simulink model "svpwm_induction_motor"  (R2023b)
settings: Solver=FixedStepAuto  StartTime=0  StopTime=2  FixedStep=1e-5  RelTol=1e-3
libraries: slpidlib x3, spsAsynchronousMachineSIUnitsLib x1, spsDCVoltageSourceLib x1, simulink x1, spsabctodq0Lib x1, spsdq0toAlphaBetaZeroLib x1, spsThreePhaseVIMeasurementLib x1, spsUniversalBridgeLib x1, spspowerguiLib x1
settings Model: Creator=朱子轩  LastModifiedBy=13571

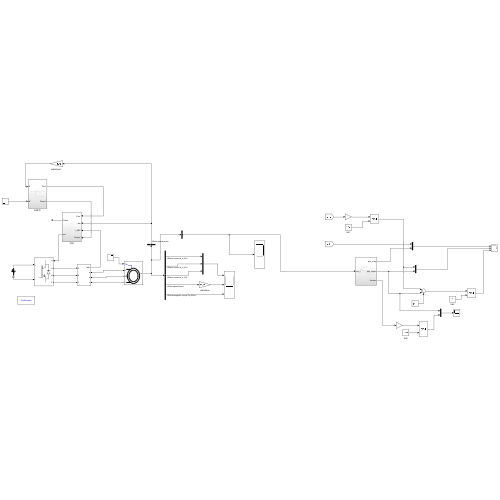
[thumbnail: Simulink's stored preview of the top-level diagram]
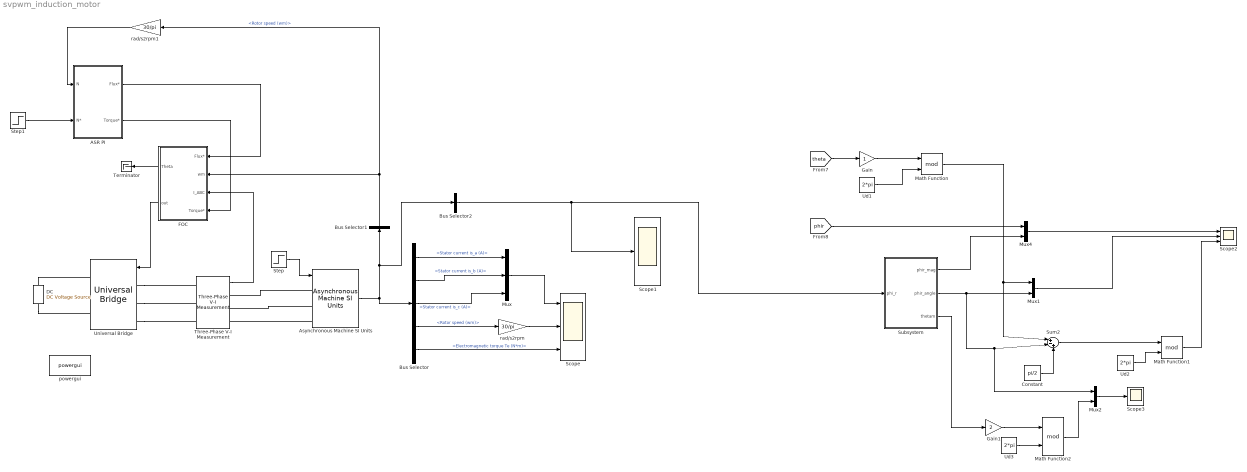
== system svpwm_induction_motor ==
  ASR PI : Subsystem
  Asynchronous Machine SI Units : spsAsynchronousMachineSIUnitsLib/Asynchronous Machine SI Units  RotorType=Squirrel-cage  PresetModel=No  MechanicalLoad=Torque Tm  ShowDetailedParameters=on  ReferenceFrame=Stationary  Units=SI  MeasurementBus=off  NominalParameters=[7500,380,50]  VoltageRatio=1  Stator=[0.7384,0.003045]  Rotor=[0.7402,0.003045]  Cage1=[0.4155 0.002066]  Cage2=[0.4168 0.0003495]  Lm=0.1241  Mechanical=[0.0343,0,2]  PolePairs=2  InitialConditions=[1,0,0,0,0,0,0,0]  SimulateSaturation=off  Saturation=[14.03593122, 27.81365428, 53.79336849, 72.68890987, 97.98006896, 148.6815601, 215.7428561, 302.9841135, 428.7778367 ; 230, 322, 414, 460, 506, 552, 598, 644, 690]  LoadFlowParameters=1492000  TsPowergui=0  TsBlock=-1  IterativeModel=Trapezoidal non iterative  IterativeDiscreteModel=Trapezoidal non iterative  Pmec=1.492e+006
  Bus Selector : BusSelector  OutputSignals=Stator measurements.Stator current is_a (A),Stator measurements.Stator current is_b (A),Stator measurements.Stator current is_c (A),Mechanical.Rotor speed (wm),Mechanical.Electromagnetic torque Te (N*m)
  Bus Selector1 : BusSelector  OutputSignals=Mechanical.Rotor speed (wm)
  Bus Selector2 : BusSelector  OutputSignals=Rotor measurements.Rotor flux phir_d (V s),Rotor measurements.Rotor flux phir_q (V s),Mechanical.Rotor angle thetam (rad)  OutputAsBus=on
  Constant : Constant  Value=pi/2
  DC : spsDCVoltageSourceLib/DC Voltage Source  Amplitude=800  Measurements=None
  FOC : Subsystem
  Gain : Gain
  Gain1 : Gain  Gain=2
  Math Function : Math  Operator=mod
  Math Function1 : Math  Operator=mod
  Math Function2 : Math  Operator=mod
  Mux : Mux  Inputs=3
  Mux1 : Mux  Inputs=2
  Mux2 : Mux  Inputs=2
  Mux4 : Mux  Inputs=2
  Scope : Scope  NumInputPorts=3
  Scope1 : Scope
  Scope2 : Scope  NumInputPorts=3
  Scope3 : Scope
  Step : Step  Time=0.5  After=40  SampleTime=0
  Step1 : Step  Before=1000  After=1400  SampleTime=0
  Subsystem : Subsystem
  Sum2 : Sum  Inputs=|+-+
  Terminator : Terminator
  Three-Phase V-I Measurement : spsThreePhaseVIMeasurementLib/Three-Phase V-I Measurement  VoltageMeasurement=no  SetLabelV=off  LabelV=Vabc  Vpu=off  VpuLL=off  CurrentMeasurement=yes  SetLabelI=off  LabelI=Iabc  Ipu=off  Pbase=100e6  Vbase=500e3  OutputType=Complex  PhasorSimulation=off  PSBequivalent=0
  Ud1 : Constant  Value=2*pi
  Ud2 : Constant  Value=2*pi
  Ud3 : Constant  Value=2*pi
  Universal Bridge : spsUniversalBridgeLib/Universal Bridge  Arms=3  SnubberResistance=1e5  SnubberCapacitance=inf  Device=IGBT / Diodes  Ron=1e-3  Lon=0  ForwardVoltages="[  0  0  ]"  ForwardVoltage=0  GTOparameters=[ 10e-6 , 20e-6 ]  IGBTparameters=[ 1e-6 , 2e-6 ]  Measurements=None  Measurements_2=None  converterType=Rectifier
  powergui : spspowerguiLib/powergui  Priority=1  SimulationMode=Continuous  SampleTime=50e-6  frequency=60  Iterations=50  frequencyindice=50  Pbase=100e6  ErrMax=1e-4  UnitsV=kV  UnitsW=MW  buscounter=0  FunctionMessages=off  echomessages=off  EnableUseOfTLC=off  CurrentSourceSwitches=off  DisableSnubberDevices=off  DisableRonSwitches=off  DisableVfSwitches=off  DisplayEquations=off  AutomaticDiscreteSolvers=off  SolverType=Tustin/Backward Euler (TBE)  Interpol=off  ExternalGateDelay=off  methode=off  Ts=100  x0status=blocks  SPID=on  SwTol=0  HookPort=off  NonlinearTolerance=1e-4  nMaxIteration=100  ContinueOnMaxIteration=off  RestoreLinks=warning  ResistiveCurrentMeasurement=off  Frange=[0:2:500]  Ylog=off  Xlog=on  ShowGrid=off  save=off  variable=ZData  structure=0  ZoomFFT=off  StartTime=0.0  cycles=1  DisplayStyle=1  fundamental=60  FreqAxis=off  MaxFrequency=1000  frequencyindicesteady=1  RmsSteady=1  display=off
  rad/s2rpm : Gain  Gain=30/pi
  rad/s2rpm1 : Gain  Gain=30/pi
  wires:
  Step/1 -> Asynchronous Machine SI Units/1
  Asynchronous Machine SI Units/1 -> Bus Selector/1, Bus Selector2/1, Bus Selector1/1
  Bus Selector/1 -> Mux/1  "<Stator current is_a (A)>"
  Bus Selector/2 -> Mux/2  "<Stator current is_b (A)>"
  Bus Selector/3 -> Mux/3  "<Stator current is_c (A)>"
  Bus Selector/4 -> rad/s2rpm/1  "<Rotor speed (wm)>"
  Mux/1 -> Scope/1
  rad/s2rpm/1 -> Scope/2
  Step1/1 -> ASR PI/2(N*)
  Bus Selector1/1 -> FOC/2(wm), rad/s2rpm1/1  "<Rotor speed (wm)>"
  rad/s2rpm1/1 -> ASR PI/1(N)
  Three-Phase V-I Measurement/1 -> FOC/3(I_ABC)
  ASR PI/2(Torque*) -> FOC/4(Torque*)
  ASR PI/1(Flux*) -> FOC/1(Flux*)
  FOC/2(out) -> Universal Bridge/1
  Bus Selector2/1 -> Subsystem/1(phi_r), Scope1/1
  Bus Selector/5 -> Scope/3  "<Electromagnetic torque Te (N*m)>"
  FOC/1(Theta) -> Terminator/1
  Ud1/1 -> Math Function/2
  Ud2/1 -> Math Function1/2
  Sum2/1 -> Math Function1/1
  Subsystem/1(phir_mag) -> Mux4/2
  Gain1/1 -> Math Function2/1
  Ud3/1 -> Math Function2/2
  Gain/1 -> Math Function/1
  Mux2/1 -> Scope3/1
  Math Function2/1 -> Mux2/2
  Constant/1 -> Sum2/3
  [theta] -> Gain/1
  [phir] -> Mux4/1
  Mux4/1 -> Scope2/1
  Mux1/1 -> Scope2/2
  Subsystem/2(phir_angle) -> Mux1/2, Mux2/1, Sum2/2
  Subsystem/3(thetam) -> Gain1/1
  Math Function/1 -> Mux1/1, Sum2/1
  Math Function1/1 -> Scope2/3
  connections:
  DC/RConn1 -- Universal Bridge/RConn1
  Universal Bridge/LConn1 -- Three-Phase V-I Measurement/LConn1
  Universal Bridge/LConn2 -- Three-Phase V-I Measurement/LConn2
  Universal Bridge/LConn3 -- Three-Phase V-I Measurement/LConn3
  Asynchronous Machine SI Units/LConn3 -- Three-Phase V-I Measurement/RConn3
  Asynchronous Machine SI Units/LConn2 -- Three-Phase V-I Measurement/RConn2
  Asynchronous Machine SI Units/LConn1 -- Three-Phase V-I Measurement/RConn1
  DC/LConn1 -- Universal Bridge/RConn2

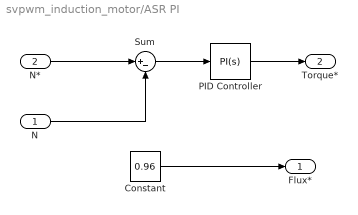
== system svpwm_induction_motor/ASR PI ==
  N : Inport
  N* : Inport  Port=2
  Constant : Constant  Value=0.96
  PID Controller : slpidlib/PID Controller  Controller=PI  Form=Parallel  TimeDomain=Continuous-time  UseExternalTs=off  SampleTime=-1  IntegratorMethod=Forward Euler  FilterMethod=Forward Euler  ControllerParametersSource=internal  P=10  I=10  UseKiTs=off  D=0  N=100  UseFilter=on  TunerSelectOption=Transfer Function Based (PID Tuner App)  InitialConditionSource=internal  InitialConditionForIntegrator=0  InitialConditionForFilter=0  DifferentiatorICPrevScaledInput=0  ExternalReset=none  TrackingMode=off  Kt=1  LimitOutput=on  SatLimitsSource=internal  UpperSaturationLimit=100  LowerSaturationLimit=-100  LinearizeAsGain=on  AntiWindupMode=back-calculation  Kb=1  LimitIntegrator=off  UpperIntegratorSaturationLimit=inf  LowerIntegratorSaturationLimit=-inf  POutMin=[]  POutMax=[]  IOutMin=[]  IOutMax=[]  DOutMin=[]  DOutMax=[]  NOutMin=[]  NOutMax=[]  SumOutMin=[]  SumOutMax=[]  SaturationOutMin=[]  SaturationOutMax=[]  PParamMin=[]  PParamMax=[]  IParamMin=[]  IParamMax=[]  DParamMin=[]  DParamMax=[]  NParamMin=[]  NParamMax=[]  KbParamMin=[]  KbParamMax=[]  KtParamMin=[]  KtParamMax=[]  KbOutMin=[]  KbOutMax=[]  KtOutMin=[]  KtOutMax=[]  IntegratorOutMin=[]  IntegratorOutMax=[]  FilterOutMin=[]  FilterOutMax=[]  SumI1OutMin=[]  SumI1OutMax=[]  SumI2OutMin=[]  SumI2OutMax=[]  SumI3OutMin=[]  SumI3OutMax=[]  SumI4OutMin=[]  SumI4OutMax=[]  SumDOutMin=[]  SumDOutMax=[]  DifferentiatorOutMin=[]  DifferentiatorOutMax=[]  FilterDiffOutCoefMin=[]  FilterDiffOutCoefMax=[]  ReciprocalOutMin=[]  ReciprocalOutMax=[]  SumDenOutMin=[]  SumDenOutMax=[]  SumNumOutMin=[]  SumNumOutMax=[]  DivideOutMin=[]  DivideOutMax=[]  UdiffTsProdOutMin=[]  UdiffTsProdOutMax=[]  NTsProdOutMin=[]  NTsProdOutMax=[]  UintegralTsProdOutMin=[]  UintegralTsProdOutMax=[]  UngainTsProdOutMin=[]  UngainTsProdOutMax=[]  ClampingZeroOutDataTypeStr=Inherit: Inherit via back propagation  ClampingZeroOutMin=[]  ClampingZeroOutMax=[]  FilterDenConstantOutDataTypeStr=Inherit: Inherit via back propagation  FilterDenConstantOutMin=[]  FilterDenConstantOutMax=[]  PCopyOutDataTypeStr=Inherit: Inherit via back propagation  PCopyOutMin=[]  PCopyOutMax=[]  NCopyOutDataTypeStr=Inherit: Inherit via back propagation  NCopyOutMin=[]  NCopyOutMax=[]  IntegratorContinuousStateAttributes=''  IntegratorStateMustResolveToSignalObject=off  IntegratorRTWStateStorageClass=Auto  FilterContinuousStateAttributes=''  FilterStateMustResolveToSignalObject=off  FilterRTWStateStorageClass=Auto  ParallelPVariant=InternalParameters  IdealPVariant=Disabled  IVariant=InternalParameters  DVariant=Disabled  IntegratorVariant=Continuous  SatVariant=Enabled  AWVariant=BackCalculation  PCopyVariant=Disabled  TRVariant=Disabled  FdbkBlocksVariant=Forward  IdealPFdbkVariant=Disabled  SatFdbkVariant=Disabled  DerivativeFilterVariant=Disabled  NVariant=Disabled  NCopyVariant=Disabled_SignalSpec  FilterICVariant=Disabled  IntegratorICVariant=InternalICs  ExternalResetVariant=Disabled  TRSumVariant=Passthrough  SumFdbkVariant=Disabled  SumVariant=Sum_PI  TsampFilterVariant=InternalTs  TsampNgainVariant=Passthrough  TsampIntegralVariant=Disabled_SignalSpec  ExternalSaturationOutDataTypeStr=Inherit: Same as second input
  Sum : Sum  Inputs=|+-
  Flux* : Outport
  Torque* : Outport  Port=2
  wires:
  N*/1 -> Sum/1
  N/1 -> Sum/2
  Constant/1 -> Flux*/1
  Sum/1 -> PID Controller/1
  PID Controller/1 -> Torque*/1

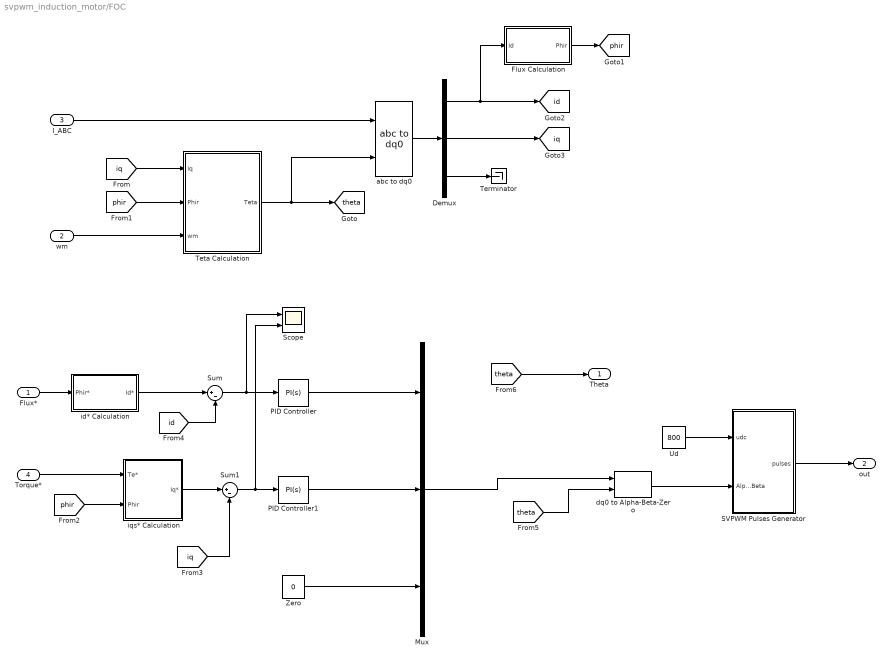
== system svpwm_induction_motor/FOC ==
  Flux* : Inport
  wm : Inport  Port=2
  I_ABC : Inport  Port=3
  Torque* : Inport  Port=4
  Demux : Demux  Outputs=3
  Flux Calculation : Subsystem
  Mux : Mux  Inputs=3
  PID Controller : slpidlib/PID Controller  Controller=PI  Form=Parallel  TimeDomain=Continuous-time  UseExternalTs=off  SampleTime=-1  IntegratorMethod=Forward Euler  FilterMethod=Forward Euler  ControllerParametersSource=internal  P=100  I=1  UseKiTs=off  D=0  N=100  UseFilter=on  TunerSelectOption=Transfer Function Based (PID Tuner App)  InitialConditionSource=internal  InitialConditionForIntegrator=0  InitialConditionForFilter=0  DifferentiatorICPrevScaledInput=0  ExternalReset=none  TrackingMode=off  Kt=1  LimitOutput=off  SatLimitsSource=internal  UpperSaturationLimit=100  LowerSaturationLimit=-100  LinearizeAsGain=on  AntiWindupMode=back-calculation  Kb=1  LimitIntegrator=off  UpperIntegratorSaturationLimit=inf  LowerIntegratorSaturationLimit=-inf  POutMin=[]  POutMax=[]  IOutMin=[]  IOutMax=[]  DOutMin=[]  DOutMax=[]  NOutMin=[]  NOutMax=[]  SumOutMin=[]  SumOutMax=[]  SaturationOutMin=[]  SaturationOutMax=[]  PParamMin=[]  PParamMax=[]  IParamMin=[]  IParamMax=[]  DParamMin=[]  DParamMax=[]  NParamMin=[]  NParamMax=[]  KbParamMin=[]  KbParamMax=[]  KtParamMin=[]  KtParamMax=[]  KbOutMin=[]  KbOutMax=[]  KtOutMin=[]  KtOutMax=[]  IntegratorOutMin=[]  IntegratorOutMax=[]  FilterOutMin=[]  FilterOutMax=[]  SumI1OutMin=[]  SumI1OutMax=[]  SumI2OutMin=[]  SumI2OutMax=[]  SumI3OutMin=[]  SumI3OutMax=[]  SumI4OutMin=[]  SumI4OutMax=[]  SumDOutMin=[]  SumDOutMax=[]  DifferentiatorOutMin=[]  DifferentiatorOutMax=[]  FilterDiffOutCoefMin=[]  FilterDiffOutCoefMax=[]  ReciprocalOutMin=[]  ReciprocalOutMax=[]  SumDenOutMin=[]  SumDenOutMax=[]  SumNumOutMin=[]  SumNumOutMax=[]  DivideOutMin=[]  DivideOutMax=[]  UdiffTsProdOutMin=[]  UdiffTsProdOutMax=[]  NTsProdOutMin=[]  NTsProdOutMax=[]  UintegralTsProdOutMin=[]  UintegralTsProdOutMax=[]  UngainTsProdOutMin=[]  UngainTsProdOutMax=[]  ClampingZeroOutDataTypeStr=Inherit: Inherit via back propagation  ClampingZeroOutMin=[]  ClampingZeroOutMax=[]  FilterDenConstantOutDataTypeStr=Inherit: Inherit via back propagation  FilterDenConstantOutMin=[]  FilterDenConstantOutMax=[]  PCopyOutDataTypeStr=Inherit: Inherit via back propagation  PCopyOutMin=[]  PCopyOutMax=[]  NCopyOutDataTypeStr=Inherit: Inherit via back propagation  NCopyOutMin=[]  NCopyOutMax=[]  IntegratorContinuousStateAttributes=''  IntegratorStateMustResolveToSignalObject=off  IntegratorRTWStateStorageClass=Auto  FilterContinuousStateAttributes=''  FilterStateMustResolveToSignalObject=off  FilterRTWStateStorageClass=Auto  ParallelPVariant=InternalParameters  IdealPVariant=Disabled  IVariant=InternalParameters  DVariant=Disabled  IntegratorVariant=Continuous  SatVariant=Disabled  AWVariant=Passthrough  PCopyVariant=Disabled  TRVariant=Disabled  FdbkBlocksVariant=Forward  IdealPFdbkVariant=Disabled  SatFdbkVariant=Disabled  DerivativeFilterVariant=Disabled  NVariant=Disabled  NCopyVariant=Disabled_SignalSpec  FilterICVariant=Disabled  IntegratorICVariant=InternalICs  ExternalResetVariant=Disabled  TRSumVariant=Passthrough  SumFdbkVariant=Disabled  SumVariant=Sum_PI  TsampFilterVariant=InternalTs  TsampNgainVariant=Passthrough  TsampIntegralVariant=Disabled_SignalSpec  ExternalSaturationOutDataTypeStr=Inherit: Same as second input
  PID Controller1 : slpidlib/PID Controller  Controller=PI  Form=Parallel  TimeDomain=Continuous-time  UseExternalTs=off  SampleTime=-1  IntegratorMethod=Forward Euler  FilterMethod=Forward Euler  ControllerParametersSource=internal  P=100  I=1  UseKiTs=off  D=0  N=100  UseFilter=on  TunerSelectOption=Transfer Function Based (PID Tuner App)  InitialConditionSource=internal  InitialConditionForIntegrator=0  InitialConditionForFilter=0  DifferentiatorICPrevScaledInput=0  ExternalReset=none  TrackingMode=off  Kt=1  LimitOutput=off  SatLimitsSource=internal  UpperSaturationLimit=100  LowerSaturationLimit=-100  LinearizeAsGain=on  AntiWindupMode=back-calculation  Kb=1  LimitIntegrator=off  UpperIntegratorSaturationLimit=inf  LowerIntegratorSaturationLimit=-inf  POutMin=[]  POutMax=[]  IOutMin=[]  IOutMax=[]  DOutMin=[]  DOutMax=[]  NOutMin=[]  NOutMax=[]  SumOutMin=[]  SumOutMax=[]  SaturationOutMin=[]  SaturationOutMax=[]  PParamMin=[]  PParamMax=[]  IParamMin=[]  IParamMax=[]  DParamMin=[]  DParamMax=[]  NParamMin=[]  NParamMax=[]  KbParamMin=[]  KbParamMax=[]  KtParamMin=[]  KtParamMax=[]  KbOutMin=[]  KbOutMax=[]  KtOutMin=[]  KtOutMax=[]  IntegratorOutMin=[]  IntegratorOutMax=[]  FilterOutMin=[]  FilterOutMax=[]  SumI1OutMin=[]  SumI1OutMax=[]  SumI2OutMin=[]  SumI2OutMax=[]  SumI3OutMin=[]  SumI3OutMax=[]  SumI4OutMin=[]  SumI4OutMax=[]  SumDOutMin=[]  SumDOutMax=[]  DifferentiatorOutMin=[]  DifferentiatorOutMax=[]  FilterDiffOutCoefMin=[]  FilterDiffOutCoefMax=[]  ReciprocalOutMin=[]  ReciprocalOutMax=[]  SumDenOutMin=[]  SumDenOutMax=[]  SumNumOutMin=[]  SumNumOutMax=[]  DivideOutMin=[]  DivideOutMax=[]  UdiffTsProdOutMin=[]  UdiffTsProdOutMax=[]  NTsProdOutMin=[]  NTsProdOutMax=[]  UintegralTsProdOutMin=[]  UintegralTsProdOutMax=[]  UngainTsProdOutMin=[]  UngainTsProdOutMax=[]  ClampingZeroOutDataTypeStr=Inherit: Inherit via back propagation  ClampingZeroOutMin=[]  ClampingZeroOutMax=[]  FilterDenConstantOutDataTypeStr=Inherit: Inherit via back propagation  FilterDenConstantOutMin=[]  FilterDenConstantOutMax=[]  PCopyOutDataTypeStr=Inherit: Inherit via back propagation  PCopyOutMin=[]  PCopyOutMax=[]  NCopyOutDataTypeStr=Inherit: Inherit via back propagation  NCopyOutMin=[]  NCopyOutMax=[]  IntegratorContinuousStateAttributes=''  IntegratorStateMustResolveToSignalObject=off  IntegratorRTWStateStorageClass=Auto  FilterContinuousStateAttributes=''  FilterStateMustResolveToSignalObject=off  FilterRTWStateStorageClass=Auto  ParallelPVariant=InternalParameters  IdealPVariant=Disabled  IVariant=InternalParameters  DVariant=Disabled  IntegratorVariant=Continuous  SatVariant=Disabled  AWVariant=Passthrough  PCopyVariant=Disabled  TRVariant=Disabled  FdbkBlocksVariant=Forward  IdealPFdbkVariant=Disabled  SatFdbkVariant=Disabled  DerivativeFilterVariant=Disabled  NVariant=Disabled  NCopyVariant=Disabled_SignalSpec  FilterICVariant=Disabled  IntegratorICVariant=InternalICs  ExternalResetVariant=Disabled  TRSumVariant=Passthrough  SumFdbkVariant=Disabled  SumVariant=Sum_PI  TsampFilterVariant=InternalTs  TsampNgainVariant=Passthrough  TsampIntegralVariant=Disabled_SignalSpec  ExternalSaturationOutDataTypeStr=Inherit: Same as second input
  SVPWM Pulses Generator : Subsystem
  Scope : Scope  NumInputPorts=2
  Sum : Sum  Inputs=|+-
  Sum1 : Sum  Inputs=|+-
  Terminator : Terminator
  Teta Calculation : Subsystem
  Ud : Constant  Value=800
  Zero : Constant  Value=0  OutDataTypeStr=Inherit: Inherit via back propagation
  abc to dq0 : spsabctodq0Lib/abc to dq0  Alignment=Aligned with phase A axis
  dq0 to Alpha-Beta-Zero : spsdq0toAlphaBetaZeroLib/dq0 to Alpha-Beta-Zero  Alignment=Aligned with phase A axis
  id* Calculation : Subsystem
  iqs* Calculation : Subsystem
  Theta : Outport
  out : Outport  Port=2
  tag scope: id=global, iq=global, phir=global, theta=global
  wires:
  I_ABC/1 -> abc to dq0/1
  abc to dq0/1 -> Demux/1
  Demux/1 -> Flux Calculation/1(Id), [id]
  Demux/2 -> [iq]
  Demux/3 -> Terminator/1
  [iq] -> Teta Calculation/1(Iq)
  [phir] -> Teta Calculation/2(Phir)
  Teta Calculation/1(Teta) -> abc to dq0/2, [theta]
  wm/1 -> Teta Calculation/3(wm)
  Flux Calculation/1(Phir) -> [phir]
  [phir] -> iqs* Calculation/2(Phir)
  Torque*/1 -> iqs* Calculation/1(Te*)
  Flux*/1 -> id* Calculation/1(Phir*)
  id* Calculation/1(Id*) -> Sum/1
  Sum/1 -> Scope/1, PID Controller/1
  [id] -> Sum/2
  iqs* Calculation/1(Iq*) -> Sum1/1
  Sum1/1 -> Scope/2, PID Controller1/1
  [iq] -> Sum1/2
  PID Controller1/1 -> Mux/2
  PID Controller/1 -> Mux/1
  Zero/1 -> Mux/3
  [theta] -> dq0 to Alpha-Beta-Zero/2
  Mux/1 -> dq0 to Alpha-Beta-Zero/1
  [theta] -> Theta/1
  dq0 to Alpha-Beta-Zero/1 -> SVPWM Pulses Generator/2(Alpha-Beta)
  Ud/1 -> SVPWM Pulses Generator/1(udc)
  SVPWM Pulses Generator/1(pulses) -> out/1

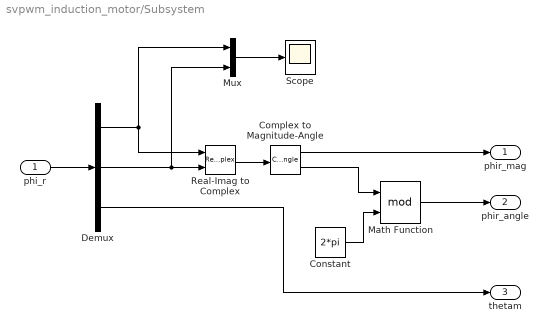
== system svpwm_induction_motor/Subsystem ==
  phi_r : Inport
  Complex to Magnitude-Angle : ComplexToMagnitudeAngle
  Constant : Constant  Value=2*pi
  Demux : Demux  Outputs=3
  Math Function : Math  Operator=mod
  Mux : Mux  Inputs=2
  Real-Imag to Complex : RealImagToComplex
  Scope : Scope
  phir_mag : Outport
  phir_angle : Outport  Port=2
  thetam : Outport  Port=3
  wires:
  phi_r/1 -> Demux/1
  Real-Imag to Complex/1 -> Complex to Magnitude-Angle/1
  Demux/2 -> Mux/2, Real-Imag to Complex/2
  Demux/1 -> Mux/1, Real-Imag to Complex/1
  Mux/1 -> Scope/1
  Demux/3 -> thetam/1
  Complex to Magnitude-Angle/1 -> phir_mag/1
  Complex to Magnitude-Angle/2 -> Math Function/1
  Constant/1 -> Math Function/2
  Math Function/1 -> phir_angle/1

== system svpwm_induction_motor/FOC/Flux Calculation ==
  Id : Inport
  Lm : Gain  Gain=0.1241
  Transfer Fcn : TransferFcn  Denominator=[0.17177 1]
  Phir : Outport
  wires:
  Id/1 -> Lm/1
  Lm/1 -> Transfer Fcn/1
  Transfer Fcn/1 -> Phir/1

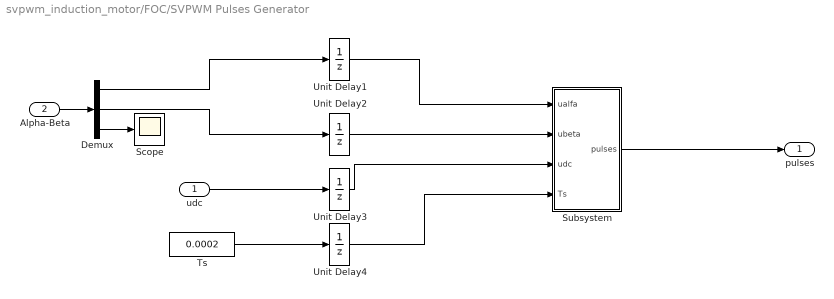
== system svpwm_induction_motor/FOC/SVPWM Pulses Generator ==
  udc : Inport
  Alpha-Beta : Inport  Port=2
  Demux : Demux  Outputs=3
  Scope : Scope
  Subsystem : Subsystem
  Ts : Constant  Value=0.0002
  Unit Delay{1..4} (4 alike) : UnitDelay  InitialCondition=5e-6  SampleTime=-1  HasFrameUpgradeWarning=on
  pulses : Outport
  wires:
  Subsystem/1(pulses) -> pulses/1
  Demux/1 -> Unit Delay1/1
  Demux/2 -> Unit Delay2/1
  udc/1 -> Unit Delay3/1
  Ts/1 -> Unit Delay4/1
  Unit Delay4/1 -> Subsystem/4(Ts)
  Unit Delay3/1 -> Subsystem/3(udc)
  Unit Delay2/1 -> Subsystem/2(ubeta)
  Unit Delay1/1 -> Subsystem/1(ualfa)
  Alpha-Beta/1 -> Demux/1
  Demux/3 -> Scope/1

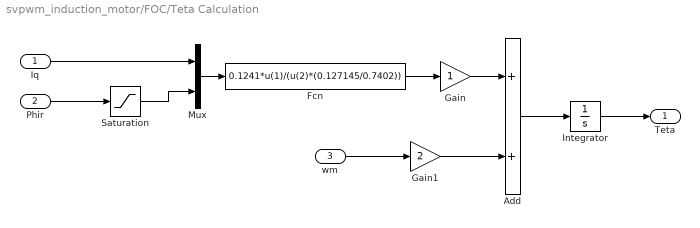
== system svpwm_induction_motor/FOC/Teta Calculation ==
  Iq : Inport
  Phir : Inport  Port=2
  wm : Inport  Port=3
  Add : Sum
  Fcn : Fcn  Expr=0.1241*u(1)/(u(2)*(0.127145/0.7402))
  Gain : Gain
  Gain1 : Gain  Gain=2
  Integrator : Integrator
  Mux : Mux  Inputs=2
  Saturation : Saturate  UpperLimit=inf  LowerLimit=1e-3
  Teta : Outport
  wires:
  Phir/1 -> Saturation/1
  Iq/1 -> Mux/1
  Add/1 -> Integrator/1
  Integrator/1 -> Teta/1
  Fcn/1 -> Gain/1
  Gain/1 -> Add/1
  wm/1 -> Gain1/1
  Gain1/1 -> Add/2
  Mux/1 -> Fcn/1
  Saturation/1 -> Mux/2

== system svpwm_induction_motor/FOC/id* Calculation ==
  Phir* : Inport
  KF : Gain  Gain=1/0.1241
  Id* : Outport
  wires:
  Phir*/1 -> KF/1
  KF/1 -> Id*/1

== system svpwm_induction_motor/FOC/iqs* Calculation ==
  Te* : Inport
  Phir : Inport  Port=2
  Fcn : Fcn  Expr=(2/3)*(1/2)*(0.127145/0.1241)*u[1]/(u[2])
  Mux : Mux  Inputs=2
  Saturation : Saturate  UpperLimit=inf  LowerLimit=1e-3
  Iq* : Outport
  wires:
  Phir/1 -> Saturation/1
  Fcn/1 -> Iq*/1
  Saturation/1 -> Mux/2
  Te*/1 -> Mux/1
  Mux/1 -> Fcn/1

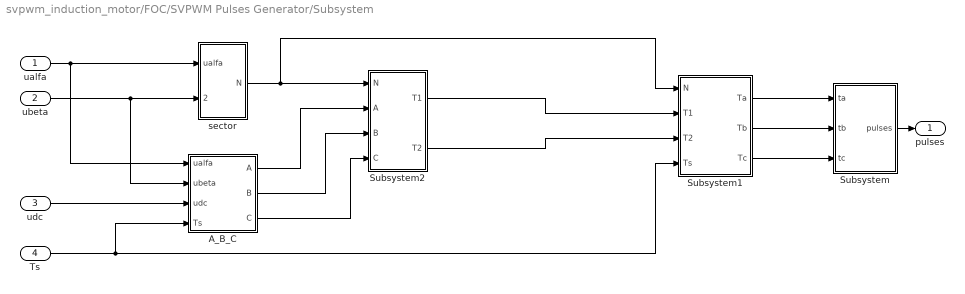
== system svpwm_induction_motor/FOC/SVPWM Pulses Generator/Subsystem ==
  ualfa : Inport
  ubeta : Inport  Port=2
  udc : Inport  Port=3
  Ts : Inport  Port=4
  A_B_C : Subsystem
  Subsystem : Subsystem
  Subsystem1 : Subsystem
  Subsystem2 : Subsystem
  sector : Subsystem
  pulses : Outport
  wires:
  A_B_C/1(A) -> Subsystem2/2(A)
  A_B_C/2(B) -> Subsystem2/3(B)
  A_B_C/3(C) -> Subsystem2/4(C)
  Subsystem1/1(Ta) -> Subsystem/1(ta)
  Subsystem1/2(Tb) -> Subsystem/2(tb)
  Subsystem1/3(Tc) -> Subsystem/3(tc)
  ualfa/1 -> A_B_C/1(ualfa), sector/1(ualfa)
  udc/1 -> A_B_C/3(udc)
  Ts/1 -> Subsystem1/4(Ts), A_B_C/4(Ts)
  Subsystem/1(pulses) -> pulses/1
  sector/1(N) -> Subsystem2/1(N), Subsystem1/1(N)
  ubeta/1 -> sector/2(ubeta), A_B_C/2(ubeta)
  Subsystem2/1(T1) -> Subsystem1/2(T1)
  Subsystem2/2(T2) -> Subsystem1/3(T2)

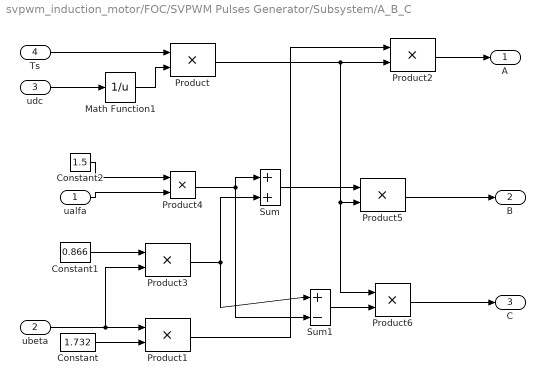
== system svpwm_induction_motor/FOC/SVPWM Pulses Generator/Subsystem/A_B_C ==
  ualfa : Inport
  ubeta : Inport  Port=2
  udc : Inport  Port=3
  Ts : Inport  Port=4
  Constant : Constant  Value=1.732
  Constant1 : Constant  Value=0.866
  Constant2 : Constant  Value=1.5
  Math Function1 : Math  Operator=reciprocal  SignedPower=on
  Product{,1..6} (7 alike) : Product  SaturateOnIntegerOverflow=on  OutDataTypeStr=Inherit: Same as first input
  Sum : Sum  Inputs=|++  SaturateOnIntegerOverflow=on
  Sum1 : Sum  Inputs=|+-  SaturateOnIntegerOverflow=on
  A : Outport
  B : Outport  Port=2
  C : Outport  Port=3
  wires:
  udc/1 -> Math Function1/1
  Ts/1 -> Product/1
  Math Function1/1 -> Product/2
  ubeta/1 -> Product1/1, Product3/2
  Constant/1 -> Product1/2
  Product1/1 -> Product2/1
  Constant1/1 -> Product3/1
  Constant2/1 -> Product4/1
  ualfa/1 -> Product4/2
  Product4/1 -> Sum/1, Sum1/2
  Product3/1 -> Sum/2, Sum1/1
  Sum/1 -> Product5/1
  Product/1 -> Product2/2, Product5/2, Product6/1
  Product2/1 -> A/1
  Product5/1 -> B/1
  Sum1/1 -> Product6/2
  Product6/1 -> C/1

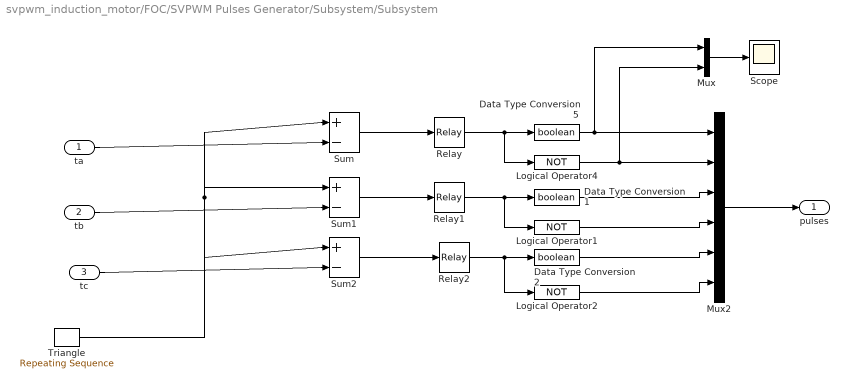
== system svpwm_induction_motor/FOC/SVPWM Pulses Generator/Subsystem/Subsystem ==
  ta : Inport
  tb : Inport  Port=2
  tc : Inport  Port=3
  Data Type Conversion1 : DataTypeConversion  OutDataTypeStr=boolean
  Data Type Conversion2 : DataTypeConversion  OutDataTypeStr=boolean
  Data Type Conversion5 : DataTypeConversion  OutDataTypeStr=boolean
  Logical Operator1 : Logic  Operator=NOT  AllPortsSameDT=off
  Logical Operator2 : Logic  Operator=NOT  AllPortsSameDT=off
  Logical Operator4 : Logic  Operator=NOT  AllPortsSameDT=off
  Mux : Mux  Inputs=2
  Mux2 : Mux  Inputs=6
  Relay : Relay  OnSwitchValue=0.000000001  OffSwitchValue=-0.000000001
  Relay1 : Relay  OnSwitchValue=0.000000001  OffSwitchValue=-0.000000001
  Relay2 : Relay  OnSwitchValue=0.000000001  OffSwitchValue=-0.000000001
  Scope : Scope
  Sum : Sum  Inputs=|+-  SaturateOnIntegerOverflow=on
  Sum1 : Sum  Inputs=|+-  SaturateOnIntegerOverflow=on
  Sum2 : Sum  Inputs=|+-  SaturateOnIntegerOverflow=on
  Triangle : simulink/Sources/Repeating Sequence  rep_seq_t=[0 0.0001 0.0002]  rep_seq_y=[0 0.0001 0]
  pulses : Outport
  wires:
  Triangle/1 -> Sum/1, Sum1/1, Sum2/1
  ta/1 -> Sum/2
  tc/1 -> Sum2/2
  tb/1 -> Sum1/2
  Sum/1 -> Relay/1
  Sum1/1 -> Relay1/1
  Sum2/1 -> Relay2/1
  Mux2/1 -> pulses/1
  Relay/1 -> Data Type Conversion5/1, Logical Operator4/1
  Relay1/1 -> Data Type Conversion1/1, Logical Operator1/1
  Relay2/1 -> Data Type Conversion2/1, Logical Operator2/1
  Data Type Conversion5/1 -> Mux/1, Mux2/1
  Logical Operator4/1 -> Mux2/2, Mux/2
  Data Type Conversion2/1 -> Mux2/5
  Logical Operator2/1 -> Mux2/6
  Data Type Conversion1/1 -> Mux2/3
  Logical Operator1/1 -> Mux2/4
  Mux/1 -> Scope/1

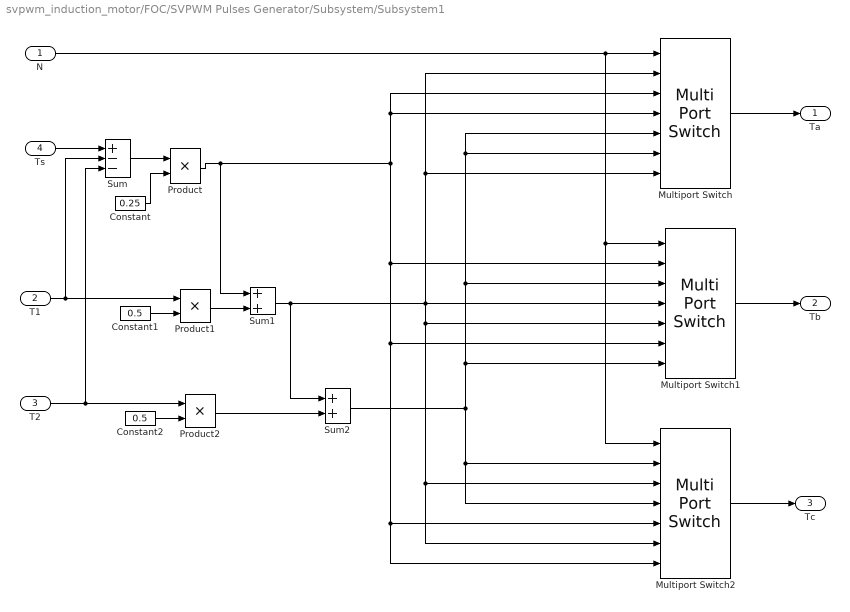
== system svpwm_induction_motor/FOC/SVPWM Pulses Generator/Subsystem/Subsystem1 ==
  N : Inport
  T1 : Inport  Port=2
  T2 : Inport  Port=3
  Ts : Inport  Port=4
  Constant : Constant  Value=0.25
  Constant1 : Constant  Value=0.5
  Constant2 : Constant  Value=0.5
  Multiport Switch : MultiPortSwitch  Inputs=6  InputSameDT=off
  Multiport Switch1 : MultiPortSwitch  Inputs=6  InputSameDT=off
  Multiport Switch2 : MultiPortSwitch  Inputs=6  InputSameDT=off
  Product : Product  SaturateOnIntegerOverflow=on  OutDataTypeStr=Inherit: Same as first input
  Product1 : Product  SaturateOnIntegerOverflow=on  OutDataTypeStr=Inherit: Same as first input
  Product2 : Product  SaturateOnIntegerOverflow=on  OutDataTypeStr=Inherit: Same as first input
  Sum : Sum  Inputs=+--  SaturateOnIntegerOverflow=on
  Sum1 : Sum  SaturateOnIntegerOverflow=on
  Sum2 : Sum  SaturateOnIntegerOverflow=on
  Ta : Outport
  Tb : Outport  Port=2
  Tc : Outport  Port=3
  wires:
  Product/1 -> Multiport Switch/3, Multiport Switch/4, Multiport Switch1/2, Multiport Switch1/6, Multiport Switch2/5, Multiport Switch2/7, Sum1/1
  Sum1/1 -> Multiport Switch1/4, Multiport Switch1/5, Multiport Switch2/3, Multiport Switch2/6, Multiport Switch/2, Multiport Switch/7, Sum2/1
  Sum2/1 -> Multiport Switch2/2, Multiport Switch2/4, Multiport Switch1/3, Multiport Switch/5, Multiport Switch/6, Multiport Switch1/7
  Multiport Switch/1 -> Ta/1
  Multiport Switch1/1 -> Tb/1
  Multiport Switch2/1 -> Tc/1
  N/1 -> Multiport Switch/1, Multiport Switch1/1, Multiport Switch2/1
  Ts/1 -> Sum/1
  T1/1 -> Sum/2, Product1/1
  T2/1 -> Sum/3, Product2/1
  Sum/1 -> Product/1
  Constant/1 -> Product/2
  Constant1/1 -> Product1/2
  Constant2/1 -> Product2/2
  Product1/1 -> Sum1/2
  Product2/1 -> Sum2/2

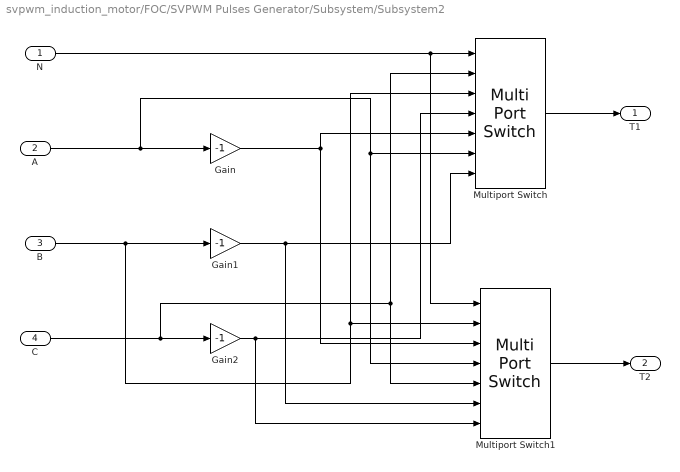
== system svpwm_induction_motor/FOC/SVPWM Pulses Generator/Subsystem/Subsystem2 ==
  N : Inport
  A : Inport  Port=2
  B : Inport  Port=3
  C : Inport  Port=4
  Gain : Gain  Gain=-1  SaturateOnIntegerOverflow=on  OutDataTypeStr=Inherit: Same as input  ParamDataTypeStr=Inherit: Same as input
  Gain1 : Gain  Gain=-1  SaturateOnIntegerOverflow=on  OutDataTypeStr=Inherit: Same as input  ParamDataTypeStr=Inherit: Same as input
  Gain2 : Gain  Gain=-1  SaturateOnIntegerOverflow=on  OutDataTypeStr=Inherit: Same as input  ParamDataTypeStr=Inherit: Same as input
  Multiport Switch : MultiPortSwitch  Inputs=6  InputSameDT=off
  Multiport Switch1 : MultiPortSwitch  Inputs=6  InputSameDT=off
  T1 : Outport
  T2 : Outport  Port=2
  wires:
  A/1 -> Gain/1, Multiport Switch1/4, Multiport Switch/6
  B/1 -> Gain1/1, Multiport Switch1/2, Multiport Switch/3
  C/1 -> Gain2/1, Multiport Switch/2, Multiport Switch1/5
  N/1 -> Multiport Switch/1, Multiport Switch1/1
  Gain/1 -> Multiport Switch1/3, Multiport Switch/5
  Gain2/1 -> Multiport Switch/4, Multiport Switch1/7
  Gain1/1 -> Multiport Switch1/6, Multiport Switch/7
  Multiport Switch/1 -> T1/1
  Multiport Switch1/1 -> T2/1

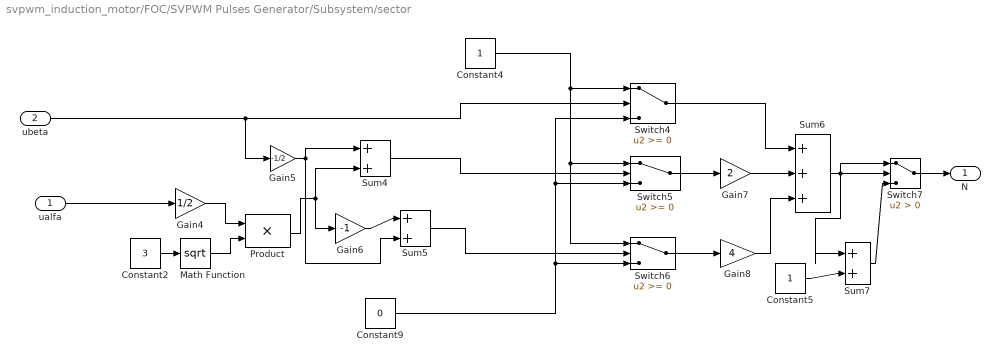
== system svpwm_induction_motor/FOC/SVPWM Pulses Generator/Subsystem/sector ==
  ualfa : Inport
  ubeta : Inport  Port=2
  Constant2 : Constant  Value=3
  Constant4 : Constant
  Constant5 : Constant
  Constant9 : Constant  Value=0
  Gain4 : Gain  Gain=1/2  SaturateOnIntegerOverflow=on  OutDataTypeStr=Inherit: Same as input  ParamDataTypeStr=Inherit: Same as input
  Gain5 : Gain  Gain=-1/2  SaturateOnIntegerOverflow=on  OutDataTypeStr=Inherit: Same as input  ParamDataTypeStr=Inherit: Same as input
  Gain6 : Gain  Gain=-1  SaturateOnIntegerOverflow=on  OutDataTypeStr=Inherit: Same as input  ParamDataTypeStr=Inherit: Same as input
  Gain7 : Gain  Gain=2  SaturateOnIntegerOverflow=on  OutDataTypeStr=Inherit: Same as input  ParamDataTypeStr=Inherit: Same as input
  Gain8 : Gain  Gain=4  SaturateOnIntegerOverflow=on  OutDataTypeStr=Inherit: Same as input  ParamDataTypeStr=Inherit: Same as input
  Math Function : Math  Operator=sqrt  SignedPower=on
  Product : Product  InputSameDT=on  SaturateOnIntegerOverflow=on  OutDataTypeStr=Inherit: Same as first input
  Sum4 : Sum  Inputs=|++  InputSameDT=on  SaturateOnIntegerOverflow=on  OutDataTypeStr=Inherit: Same as first input
  Sum5 : Sum  Inputs=|++  InputSameDT=on  SaturateOnIntegerOverflow=on  OutDataTypeStr=Inherit: Same as first input
  Sum6 : Sum  Inputs=+++  SaturateOnIntegerOverflow=on
  Sum7 : Sum  Inputs=|++  SaturateOnIntegerOverflow=on
  Switch4 : Switch
  Switch5 : Switch
  Switch6 : Switch
  Switch7 : Switch  Criteria=u2 > Threshold  InputSameDT=off
  N : Outport
  wires:
  ualfa/1 -> Gain4/1
  ubeta/1 -> Gain5/1, Switch4/2
  Gain5/1 -> Sum4/1, Sum5/2
  Product/1 -> Sum4/2, Gain6/1
  Sum4/1 -> Switch5/2
  Gain6/1 -> Sum5/1
  Sum5/1 -> Switch6/2
  Constant2/1 -> Math Function/1
  Math Function/1 -> Product/2
  Gain4/1 -> Product/1
  Switch4/1 -> Sum6/1
  Switch6/1 -> Gain8/1
  Constant9/1 -> Switch6/3, Switch4/3, Switch5/3
  Switch5/1 -> Gain7/1
  Constant4/1 -> Switch4/1, Switch6/1, Switch5/1
  Gain7/1 -> Sum6/2
  Gain8/1 -> Sum6/3
  Sum6/1 -> Switch7/2, Switch7/1, Sum7/1
  Switch7/1 -> N/1
  Sum7/1 -> Switch7/3
  Constant5/1 -> Sum7/2
